simulink model "AlgebraicLoopwithAtomic"  (R2015a)
settings: Solver=FixedStepDiscrete  SolverMode=SingleTasking  StartTime=0.0  StopTime=10.0  RelTol=1e-3
settings Model: CovMetricSettings=dwe  CovHtmlReporting=off  covSaveCumulativeToWorkspaceVar=off  CovSaveSingleToWorkspaceVar=off  CovExternalEMLEnable=on  Creator=hbourbou  LastModifiedBy=hbourbou
settings DataIOCC: LimitDataPoints=off  SaveFormat=Dataset
settings DebuggingCC: InvalidFcnCallConnMsg=warning  FcnCallInpInsideContextMsg=EnableAllAsWarning  SFUnexpectedBacktrackingDiag=error  SFNoUnconditionalDefaultTransitionDiag=error
settings HardwareCC: ProdBitPerPointer=64  ProdLargestAtomicFloat=Float  ProdIntDivRoundTo=Zero  ProdEndianess=LittleEndian  ProdHWDeviceType=Specified
settings ModelReferenceCC: PropagateSignalLabelsOutOfModel=on
settings GRTTargetCC: TargetLangStandard=C99 (ISO)  GeneratePreprocessorConditionals=Use local settings

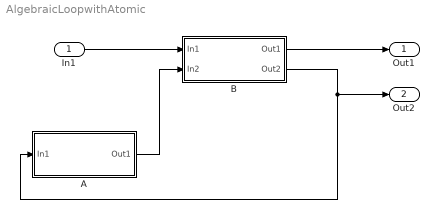
== system AlgebraicLoopwithAtomic ==
  In1 : Inport
  A : Subsystem  TreatAsAtomicUnit=on
  B : Subsystem
  Out1 : Outport
  Out2 : Outport  Port=2
  wires:
  A/1(Out1) -> B/2(In2)
  B/2(Out2) -> A/1(In1), Out2/1
  B/1(Out1) -> Out1/1
  In1/1 -> B/1(In1)

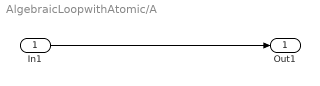
== system AlgebraicLoopwithAtomic/A ==
  In1 : Inport
  Out1 : Outport
  wires:
  In1/1 -> Out1/1

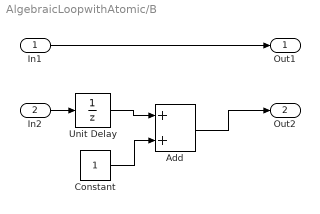
== system AlgebraicLoopwithAtomic/B ==
  In1 : Inport
  In2 : Inport  Port=2
  Add : Sum
  Constant : Constant
  Unit Delay : UnitDelay  SampleTime=-1
  Out1 : Outport
  Out2 : Outport  Port=2
  wires:
  In1/1 -> Out1/1
  Add/1 -> Out2/1
  In2/1 -> Unit Delay/1
  Unit Delay/1 -> Add/1
  Constant/1 -> Add/2
